simulink model "lab1Sim"  (R2024b)
settings: Solver=VariableStepAuto  StartTime=0.0  StopTime=10.0  MaxStep=5  RelTol=1e-3
values from neighbouring files (symbols this model uses):
  cpp = 1000    [lab1v2.m]
  Cvs = cps * ros * Vs    (= 9240000)    [lab1v2.m]
  Cvw = cpp * rop * Vw    (= 150000)    [lab1v2.m]
  czas_skok = 10000    [lab1v2.m]
  dFp = 0    [lab1v2.m]
  dPg = 0    [lab1v2.m]
  dTzew = 1    [lab1v2.m]
  Fp0 = FpN * 1.0    (= 0.0694444444444)    [lab1v2.m]
  Ks = Px/(TsN - TzewN)    (= 133.333333333)    [lab1v2.m]
  Kw = Px/(TwewN - TsN)    (= 933.333333333)    [lab1v2.m]
  Pg0 = tab_Ts(i)    [lab1v2.m]
  rop = 1.2    [lab1v2.m]
  Ts0 = (Kw*Twew0 + Ks*Tzew0) / (Kw + Ks)    (= 15)    [lab1v2.m]
  Twew0 = (Pg0 + Tzew0*(cpp*rop*Fp0 + ((Ks*Kw)/(Kw + Ks)))) / (cpp*rop*Fp0 + ((Kw * Ks)/(Kw + Ks)))    (= 20)    [lab1v2.m]
  Tzew0 = tab_Tzew(i)    [lab1v2.m]
settings Model: Creator=Michal  LastModifiedBy=Michal

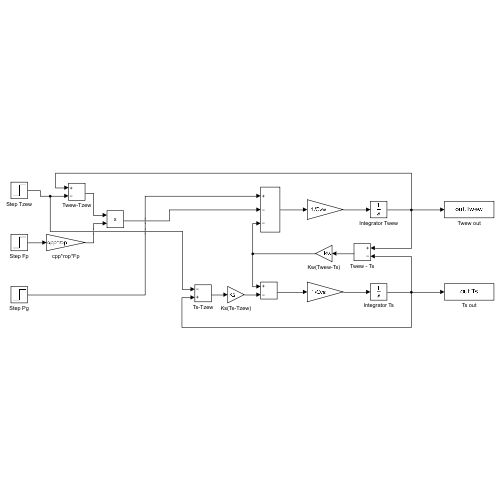
[thumbnail: Simulink's stored preview of the top-level diagram]
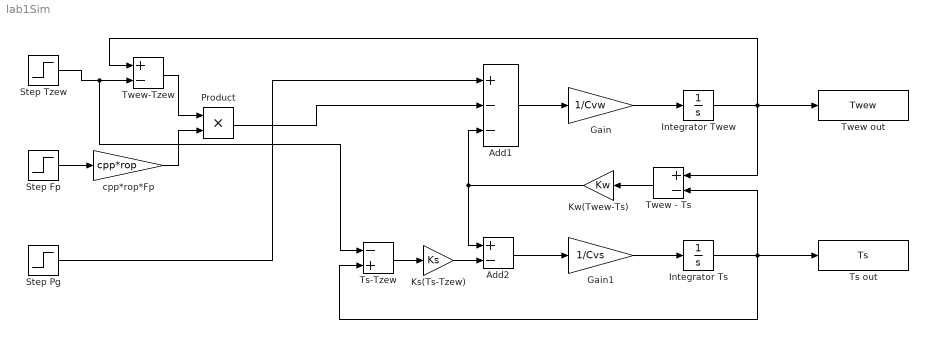
== system lab1Sim ==
  Add1 : Sum  Inputs=+--
  Add2 : Sum  Inputs=+-
  Gain : Gain  Gain=1/Cvw
  Gain1 : Gain  Gain=1/Cvs
  Integrator Ts : Integrator  InitialCondition=Ts0
  Integrator Twew : Integrator  InitialCondition=Twew0
  Ks(Ts-Tzew) : Gain  Gain=Ks
  Kw(Twew-Ts) : Gain  Gain=Kw
  Product : Product
  Step Fp : Step  Time=czas_skok  Before=Fp0  After=Fp0+dFp  SampleTime=0
  Step Pg : Step  Time=czas_skok  Before=Pg0  After=Pg0+dPg  SampleTime=0
  Step Tzew : Step  Time=czas_skok  Before=Tzew0  After=Tzew0+dTzew  SampleTime=0
  Ts out : ToWorkspace  VariableName=Ts  SampleTime=-1
  Ts-Tzew : Sum  Inputs=-+
  Twew - Ts : Sum  Inputs=+-
  Twew out : ToWorkspace  VariableName=Twew  SampleTime=-1
  Twew-Tzew : Sum  Inputs=+-
  cpp*rop*Fp : Gain  Gain=cpp*rop
  wires:
  Integrator Twew/1 -> Twew out/1, Twew-Tzew/1, Twew - Ts/1
  Integrator Ts/1 -> Ts out/1, Twew - Ts/2, Ts-Tzew/2
  Gain/1 -> Integrator Twew/1
  Gain1/1 -> Integrator Ts/1
  Add1/1 -> Gain/1
  Add2/1 -> Gain1/1
  Twew - Ts/1 -> Kw(Twew-Ts)/1
  Step Pg/1 -> Add1/1
  Kw(Twew-Ts)/1 -> Add2/1, Add1/3
  Step Tzew/1 -> Ts-Tzew/1, Twew-Tzew/2
  Step Fp/1 -> cpp*rop*Fp/1
  Twew-Tzew/1 -> Product/1
  cpp*rop*Fp/1 -> Product/2
  Product/1 -> Add1/2
  Ts-Tzew/1 -> Ks(Ts-Tzew)/1
  Ks(Ts-Tzew)/1 -> Add2/2
